simulink model "Task1"  (R2024a)
settings: Solver=VariableStepAuto  StartTime=0.0  StopTime=10.0  RelTol=1e-3
libraries: SignalEditorBlockLib x1
settings Model: Creator=mugiw  LastModifiedBy=mugiw

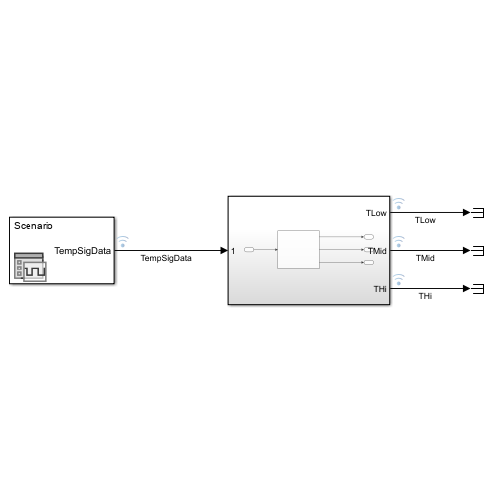
[thumbnail: Simulink's stored preview of the top-level diagram]
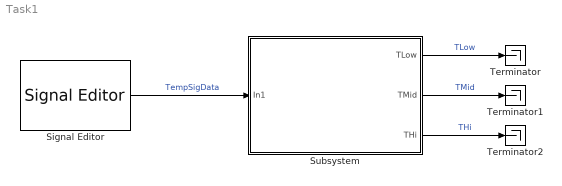
== system Task1 ==
  Signal Editor : SignalEditorBlockLib/Signal Editor  FileName=TempSignal.mat  ActiveScenario=Scenario  ActiveSignal=TempSigData  IsBus=off  OutputBusObjectStr=Bus: BusObject  SampleTime=0  Interpolate=off  ZeroCross=off  OutputAfterFinalValue=Setting to zero  Unit=inherit  PreserveSignalName=on  ApplySigPropsToAllScenarios=on  ApplySigPropsToAllSignals=off
  Subsystem : Subsystem
  Terminator : Terminator
  Terminator1 : Terminator
  Terminator2 : Terminator
  wires:
  Signal Editor/1 -> Subsystem/1(In1)  "TempSigData"
  Subsystem/2(TMid) -> Terminator1/1  "TMid"
  Subsystem/3(THi) -> Terminator2/1  "THi"
  Subsystem/1(TLow) -> Terminator/1  "TLow"

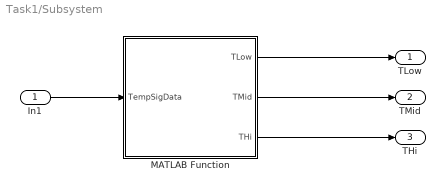
== system Task1/Subsystem ==
  In1 : Inport
  MATLAB Function : MATLAB Function  TreatAsAtomicUnit=on
  TLow : Outport
  TMid : Outport  Port=2
  THi : Outport  Port=3
  wires:
  In1/1 -> MATLAB Function/1(TempSigData)
  MATLAB Function/1(TLow) -> TLow/1
  MATLAB Function/2(TMid) -> TMid/1
  MATLAB Function/3(THi) -> THi/1

== matlab function Task1/Subsystem/MATLAB Function ==
  data: TempSigData input; TLow output; TMid output; THi output
function [TLow,TMid,THi] = fcn(TempSigData)

TLow = false;
TMid = false;
THi = false;

if(TempSigData <= 100)
    TLow = true;
elseif((TempSigData > 100) && (TempSigData <= 200))
    TMid = true;
else
    THi = true;
end
